simulink model "test_Simulink"  (R2025a)
settings: Solver=VariableStepAuto  StartTime=0.0  StopTime=10.0  RelTol=1e-3
undefined symbols (not defined in the file): A, d, F_test, k, k_m, L, l_L_0, m, mu_L, N, R, U_a
settings Model: Creator=Manuel  LastModifiedBy=Manuel

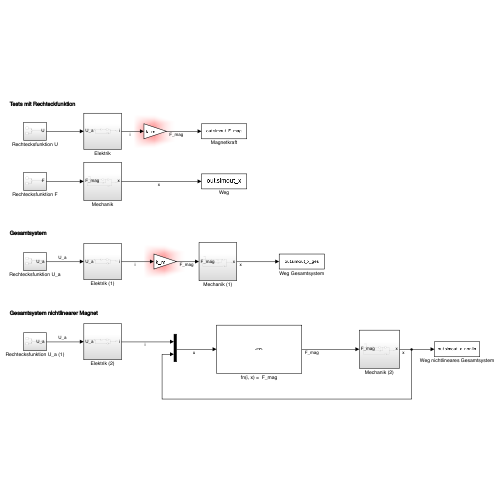
[thumbnail: Simulink's stored preview of the top-level diagram]
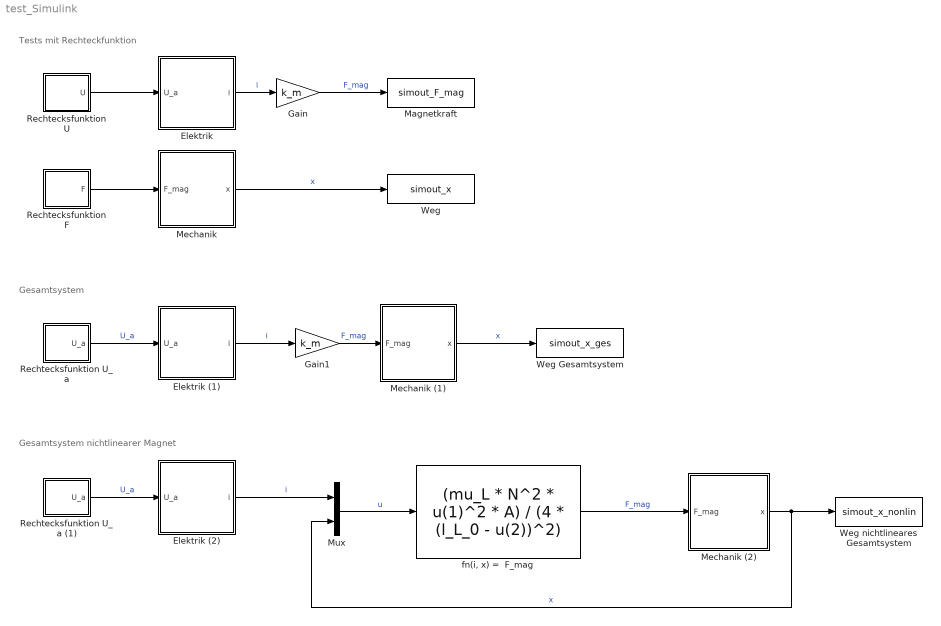
== system test_Simulink ==
  note: Gesamtsystem nichtlinearer Magnet
  note: Tests mit Rechteckfunktion
  note: Gesamtsystem
  Elektrik : Subsystem
  Elektrik (1) : Subsystem
  Elektrik (2) : Subsystem
  Gain : Gain  Gain=k_m
  Gain1 : Gain  Gain=k_m
  Magnetkraft : ToWorkspace  VariableName=simout_F_mag  SaveFormat=Structure With Time  SampleTime=-1
  Mechanik : Subsystem
  Mechanik (1) : Subsystem
  Mechanik (2) : Subsystem
  Mux : Mux  Inputs=2
  Rechtecksfunktion F : Subsystem
  Rechtecksfunktion U : Subsystem
  Rechtecksfunktion U_a : Subsystem
  Rechtecksfunktion U_a (1) : Subsystem
  Weg : ToWorkspace  VariableName=simout_x  SaveFormat=Structure With Time  SampleTime=-1
  Weg Gesamtsystem : ToWorkspace  VariableName=simout_x_ges  SaveFormat=Structure With Time  SampleTime=-1
  Weg nichtlineares Gesamtsystem : ToWorkspace  VariableName=simout_x_nonlin  SaveFormat=Structure With Time  SampleTime=-1
  "fn(i, x) =  F_mag" : MATLABFcn  MATLABFcn=(mu_L * N^2 * u(1)^2 * A) / (4 * (l_L_0 - u(2))^2)  OutputDimensions=1
  wires:
  Elektrik/1(i) -> Gain/1  "i"
  Gain1/1 -> Mechanik (1)/1(F_mag)  "F_mag"
  Mux/1 -> "fn(i, x) =  F_mag"/1  "u"
  Rechtecksfunktion U_a/1(U_a) -> Elektrik (1)/1(U_a)  "U_a"
  Rechtecksfunktion F/1(F) -> Mechanik/1(F_mag)
  Mechanik (2)/1(x) -> Mux/2, Weg nichtlineares Gesamtsystem/1  "x"
  Gain/1 -> Magnetkraft/1  "F_mag"
  Mechanik/1(x) -> Weg/1  "x"
  Rechtecksfunktion U/1(U) -> Elektrik/1(U_a)
  Elektrik (2)/1(i) -> Mux/1  "i"
  Rechtecksfunktion U_a (1)/1(U_a) -> Elektrik (2)/1(U_a)  "U_a"
  Elektrik (1)/1(i) -> Gain1/1  "i"
  "fn(i, x) =  F_mag"/1 -> Mechanik (2)/1(F_mag)  "F_mag"
  Mechanik (1)/1(x) -> Weg Gesamtsystem/1  "x"

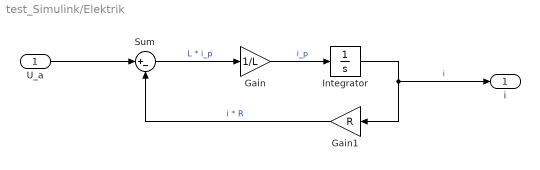
== system test_Simulink/Elektrik ==
  U_a : Inport
  Gain : Gain  Gain=1/L
  Gain1 : Gain  Gain=R
  Integrator : Integrator
  Sum : Sum  Inputs=|+-
  i : Outport
  wires:
  Integrator/1 -> i/1, Gain1/1  "i"
  Gain/1 -> Integrator/1  "i_p"
  Sum/1 -> Gain/1  "L * i_p"
  Gain1/1 -> Sum/2  "i * R"
  U_a/1 -> Sum/1

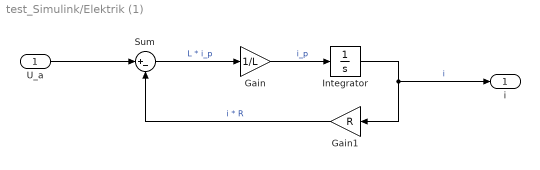
== system test_Simulink/Elektrik (1) ==
  U_a : Inport
  Gain : Gain  Gain=1/L
  Gain1 : Gain  Gain=R
  Integrator : Integrator
  Sum : Sum  Inputs=|+-
  i : Outport
  wires:
  Integrator/1 -> i/1, Gain1/1  "i"
  Gain/1 -> Integrator/1  "i_p"
  Sum/1 -> Gain/1  "L * i_p"
  Gain1/1 -> Sum/2  "i * R"
  U_a/1 -> Sum/1

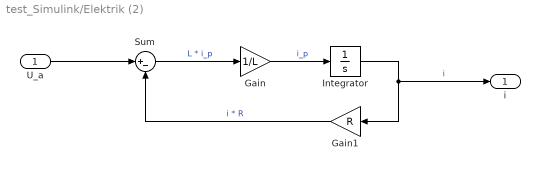
== system test_Simulink/Elektrik (2) ==
  U_a : Inport
  Gain : Gain  Gain=1/L
  Gain1 : Gain  Gain=R
  Integrator : Integrator
  Sum : Sum  Inputs=|+-
  i : Outport
  wires:
  Integrator/1 -> i/1, Gain1/1  "i"
  Gain/1 -> Integrator/1  "i_p"
  Sum/1 -> Gain/1  "L * i_p"
  Gain1/1 -> Sum/2  "i * R"
  U_a/1 -> Sum/1

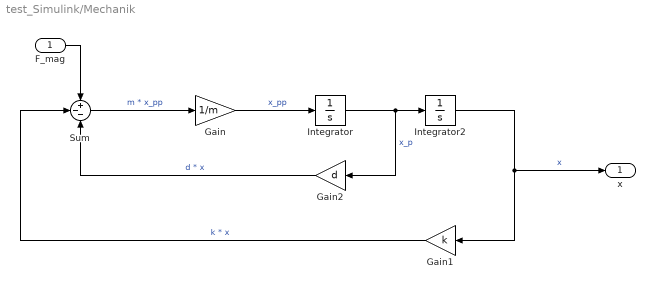
== system test_Simulink/Mechanik ==
  F_mag : Inport
  Gain : Gain  Gain=1/m
  Gain1 : Gain  Gain=k
  Gain2 : Gain  Gain=d
  Integrator : Integrator
  Integrator2 : Integrator
  Sum : Sum  Inputs=+--
  x : Outport
  wires:
  Integrator/1 -> Gain2/1, Integrator2/1  "x_p"
  Sum/1 -> Gain/1  "m * x_pp"
  Gain1/1 -> Sum/2  "k * x"
  Gain/1 -> Integrator/1  "x_pp"
  Integrator2/1 -> x/1, Gain1/1  "x"
  Gain2/1 -> Sum/3  "d * x"
  F_mag/1 -> Sum/1

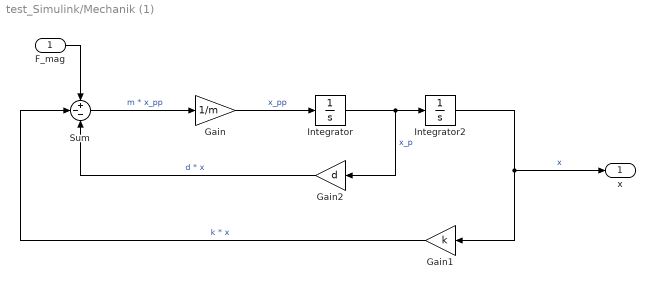
== system test_Simulink/Mechanik (1) ==
  F_mag : Inport
  Gain : Gain  Gain=1/m
  Gain1 : Gain  Gain=k
  Gain2 : Gain  Gain=d
  Integrator : Integrator
  Integrator2 : Integrator
  Sum : Sum  Inputs=+--
  x : Outport
  wires:
  Integrator/1 -> Gain2/1, Integrator2/1  "x_p"
  Sum/1 -> Gain/1  "m * x_pp"
  Gain1/1 -> Sum/2  "k * x"
  Gain/1 -> Integrator/1  "x_pp"
  Integrator2/1 -> x/1, Gain1/1  "x"
  Gain2/1 -> Sum/3  "d * x"
  F_mag/1 -> Sum/1

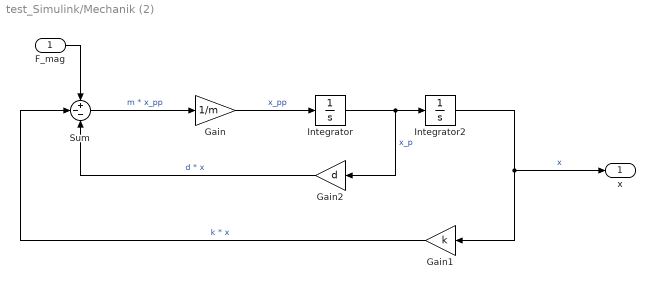
== system test_Simulink/Mechanik (2) ==
  F_mag : Inport
  Gain : Gain  Gain=1/m
  Gain1 : Gain  Gain=k
  Gain2 : Gain  Gain=d
  Integrator : Integrator
  Integrator2 : Integrator
  Sum : Sum  Inputs=+--
  x : Outport
  wires:
  Integrator/1 -> Gain2/1, Integrator2/1  "x_p"
  Sum/1 -> Gain/1  "m * x_pp"
  Gain1/1 -> Sum/2  "k * x"
  Gain/1 -> Integrator/1  "x_pp"
  Integrator2/1 -> x/1, Gain1/1  "x"
  Gain2/1 -> Sum/3  "d * x"
  F_mag/1 -> Sum/1

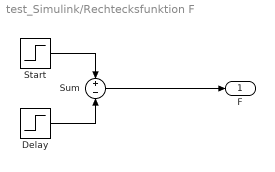
== system test_Simulink/Rechtecksfunktion F ==
  Delay : Step  Time=6  After=F_test  SampleTime=0
  Start : Step  After=F_test  SampleTime=0
  Sum : Sum  Inputs=+-
  F : Outport
  wires:
  Delay/1 -> Sum/2
  Start/1 -> Sum/1
  Sum/1 -> F/1

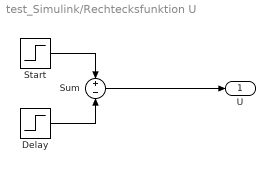
== system test_Simulink/Rechtecksfunktion U ==
  Delay : Step  Time=6  After=24  SampleTime=0
  Start : Step  After=24  SampleTime=0
  Sum : Sum  Inputs=+-
  U : Outport
  wires:
  Delay/1 -> Sum/2
  Start/1 -> Sum/1
  Sum/1 -> U/1

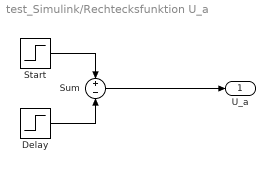
== system test_Simulink/Rechtecksfunktion U_a ==
  Delay : Step  Time=6  After=U_a  SampleTime=0
  Start : Step  After=U_a  SampleTime=0
  Sum : Sum  Inputs=+-
  U_a : Outport
  wires:
  Delay/1 -> Sum/2
  Start/1 -> Sum/1
  Sum/1 -> U_a/1

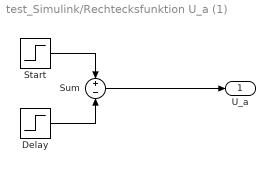
== system test_Simulink/Rechtecksfunktion U_a (1) ==
  Delay : Step  Time=6  After=U_a  SampleTime=0
  Start : Step  After=U_a  SampleTime=0
  Sum : Sum  Inputs=+-
  U_a : Outport
  wires:
  Delay/1 -> Sum/2
  Start/1 -> Sum/1
  Sum/1 -> U_a/1
